simulink model "PlasticBallMotionModel_SIM"  (R2012b)
settings: Solver=ode3  StartTime=0.0  StopTime=10.0  FixedStep=0.1  RelTol=1e-3
values from neighbouring files (symbols this model uses):
  k = 5    [PlasticBallMotionModel.m]
  v0 = v0_values(i)    [PlasticBallMotionModel.m]
settings Model: Creator=aluno  LastModifiedBy=aluno

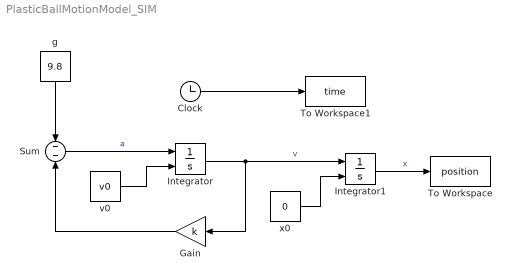
== system PlasticBallMotionModel_SIM ==
  Clock : Clock
  Gain : Gain  Gain=k
  Integrator : Integrator  InitialConditionSource=external
  Integrator1 : Integrator  InitialConditionSource=external
  Sum : Sum  Inputs=--
  To Workspace : ToWorkspace  VariableName=position  SampleTime=-1
  To Workspace1 : ToWorkspace  VariableName=time  SampleTime=-1
  g : Constant  Value=9.8
  v0 : Constant  Value=v0
  "x0 " : Constant  Value=0
  wires:
  Sum/1 -> Integrator/1  "a"
  Integrator/1 -> Integrator1/1, Gain/1  "v"
  Gain/1 -> Sum/2
  g/1 -> Sum/1
  v0/1 -> Integrator/2
  Clock/1 -> To Workspace1/1
  Integrator1/1 -> To Workspace/1  "x"
  "x0 "/1 -> Integrator1/2
